simulink model "cartPole_QFT_V2_mdl"  (R2022b)
settings: Solver=ode4  StartTime=0.0  StopTime=10  FixedStep=.001  RelTol=1e-3
undefined symbols (not defined in the file): F_x, G_theta, G_x, p_11, p_21
libraries: simulink_extras x1
settings Model: Creator=mo780715  LastModifiedBy=mo780715

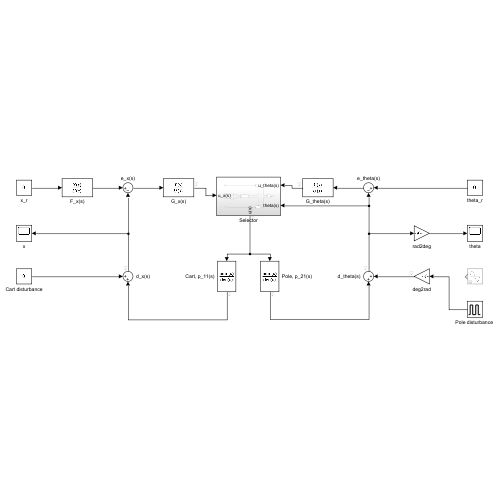
[thumbnail: Simulink's stored preview of the top-level diagram]
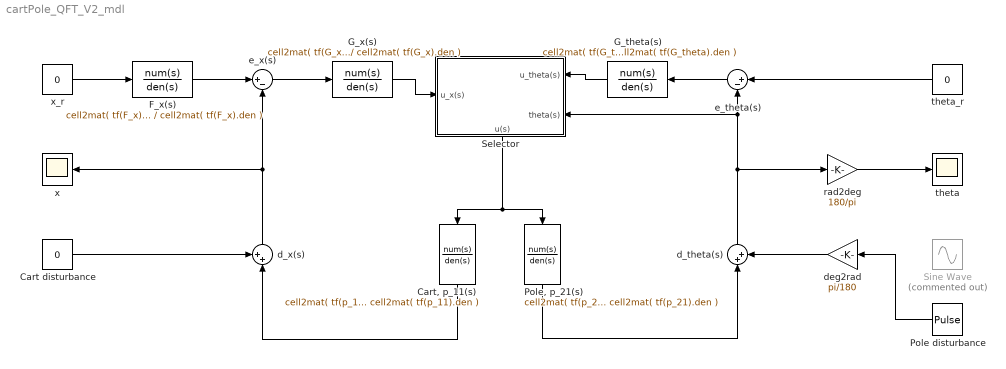
== system cartPole_QFT_V2_mdl ==
  Cart disturbance : Constant  Value=0
  "Cart, p_11(s)" : TransferFcn  Numerator=cell2mat( tf(p_11).num )  Denominator=cell2mat( tf(p_11).den )  ContinuousStateAttributes='x'
  F_x(s) : TransferFcn  Numerator=cell2mat( tf(F_x).num )  Denominator=cell2mat( tf(F_x).den )
  G_theta(s) : TransferFcn  Numerator=cell2mat( tf(G_theta).num )  Denominator=cell2mat( tf(G_theta).den )  ContinuousStateAttributes='theta'
  G_x(s) : TransferFcn  Numerator=cell2mat( tf(G_x).num )  Denominator=cell2mat( tf(G_x).den )  ContinuousStateAttributes='x'
  "Pole disturbance " : DiscretePulseGenerator  PulseType=Time based  Amplitude=-0.5  Period=100  PulseWidth=0.01  PhaseDelay=0.1
  "Pole, p_21(s)" : TransferFcn  Numerator=cell2mat( tf(p_21).num )  Denominator=cell2mat( tf(p_21).den )  ContinuousStateAttributes='theta'
  Selector : Subsystem
      settings: PortSchema="{\"entries\":[{\"content\":{\"sides\":[{\"content\":{\"connectorIds\":[\"In1\"]},\"type\":\"ConnectorPlacement.EquallySpacedRectSide\",\"uuid\":\"9fccf0fa-6994-47ef-b322-0771ca16fa7b\"},{\"content\":{\"connectorIds\":[\"In2\",\"In3\"],\"side\":\"RIGHT\"},\"type\":\"ConnectorPlacement.EquallySpacedRectSide\",\"uuid\":\"0dfb01c2-9883-4dd4-8e2a-158419bfdbc9\"},{\"content\":{\"connectorIds\":[],\"side\":\"TOP\"},\"type\":\"ConnectorPlacement.EquallySpacedRectSide\",\"uuid\":\"efb6f21b-551d-43ce-b394-b74fd7f42e11\"},{\"content\":{\"connectorIds\":[\"Out1\"],\"side\":\"BOTTOM\"},\"type\":\"ConnectorPlacement.EquallySpacedRectSide\",\"uuid\":\"ab58611c-27cd-4cec-9152-8cc366650f86\"}]},\"type\":\"ConnectorPlacement.EquallySpacedConnector\",\"uuid\":\"939a8edc-0832-4a1a-a548-ccbb7d5c0e17\"}],\"packageUris\":[\"http://schema.mathworks.com/mf0/Connector/R2020b\"],\"version\":\"1.0\"}"
  Sine Wave : Sin  Commented=on  Amplitude=0.1  SampleTime=0
  d_theta(s) : Sum  Inputs=|++
  d_x(s) : Sum  Inputs=++|
  deg2rad : Gain  Gain=pi/180
  e_theta(s) : Sum  Inputs=|+-
  e_x(s) : Sum  Inputs=|+-
  rad2deg : Gain  Gain=180/pi
  theta : Scope
  theta_r : Constant  Value=0
  x : Scope
  x_r : Constant  Value=0
  wires:
  x_r/1 -> F_x(s)/1
  "Cart, p_11(s)"/1 -> d_x(s)/2
  F_x(s)/1 -> e_x(s)/1
  theta_r/1 -> e_theta(s)/1
  e_x(s)/1 -> G_x(s)/1
  G_x(s)/1 -> Selector/1(u_x(s))
  G_theta(s)/1 -> Selector/2(u_theta(s))
  Selector/1(u(s)) -> "Cart, p_11(s)"/1, "Pole, p_21(s)"/1
  d_x(s)/1 -> x/1, e_x(s)/2
  Cart disturbance/1 -> d_x(s)/1
  deg2rad/1 -> d_theta(s)/2
  e_theta(s)/1 -> G_theta(s)/1
  "Pole, p_21(s)"/1 -> d_theta(s)/1
  d_theta(s)/1 -> rad2deg/1, e_theta(s)/2, Selector/3(theta(s))
  rad2deg/1 -> theta/1
  "Pole disturbance "/1 -> deg2rad/1

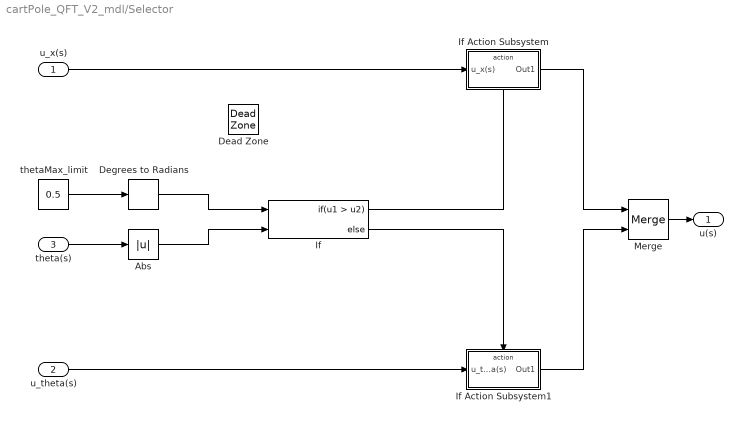
== system cartPole_QFT_V2_mdl/Selector ==
  u_x(s) : Inport
  u_theta(s) : Inport  Port=2
  theta(s) : Inport  Port=3
  Abs : Abs  SaturateOnIntegerOverflow=off
  Dead Zone : DeadZone
  Degrees to Radians : simulink_extras/Transformations/Degrees to Radians
  If : If  NumInputs=2  IfExpression=u1 > u2
  If Action Subsystem : Subsystem  TreatAsAtomicUnit=on
  If Action Subsystem1 : Subsystem  TreatAsAtomicUnit=on
  Merge : Merge
  thetaMax_limit : Constant  Value=0.5
  u(s) : Outport
  wires:
  Merge/1 -> u(s)/1
  If Action Subsystem/1(Out1) -> Merge/1
  If Action Subsystem1/1(Out1) -> Merge/2
  theta(s)/1 -> Abs/1
  u_theta(s)/1 -> If Action Subsystem1/1(u_theta(s))
  u_x(s)/1 -> If Action Subsystem/1(u_x(s))
  Abs/1 -> If/2
  thetaMax_limit/1 -> Degrees to Radians/1
  If/1 -> If Action Subsystem/Action
  If/2 -> If Action Subsystem1/Action
  Degrees to Radians/1 -> If/1

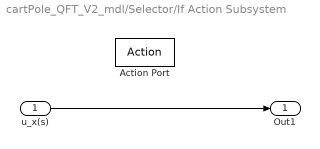
== system cartPole_QFT_V2_mdl/Selector/If Action Subsystem ==
  u_x(s) : Inport
  Action Port : ActionPort  ActionPortLabel=if(u1 > u2)
  Out1 : Outport
  wires:
  u_x(s)/1 -> Out1/1

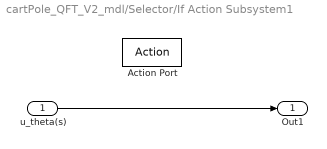
== system cartPole_QFT_V2_mdl/Selector/If Action Subsystem1 ==
  u_theta(s) : Inport
  Action Port : ActionPort  ActionPortLabel=else
  Out1 : Outport
  wires:
  u_theta(s)/1 -> Out1/1
